simulink model "ProyectoGlobal_AyCD_Cantu_LagoTejo"  (R2021a)
settings: Solver=ode23  StartTime=0.0  StopTime=inf  MinStep=1e-4
values from neighbouring files (symbols this model uses):
  a_hMax = 0.75    [Datos_ProyectoGlobal_AyCD_Cantu_LagoTejo.m]    (also in Datos_v18.m; PID_calculado.mat)
  a_tMax = 0.8    [Datos_ProyectoGlobal_AyCD_Cantu_LagoTejo.m]    (also in Datos_v18.m; PID_calculado.mat)
  b_cx = 1e6    (= 1000000)    [Datos_ProyectoGlobal_AyCD_Cantu_LagoTejo.m]    (also in Datos_v18.m; PID_calculado.mat)
  b_cy = 1e7    (= 10000000)    [Datos_ProyectoGlobal_AyCD_Cantu_LagoTejo.m]    (also in Datos_v18.m; PID_calculado.mat)
  b_eq_h = ((b_hd + b_hm*(i_h^2))*2/(r_hd^2))    (= 31004.4444444)    [Datos_ProyectoGlobal_AyCD_Cantu_LagoTejo.m]    (also in Datos_v18.m; PID_calculado.mat)
  b_eq_t = ((b_td + b_tm*(i_t^2))/(r_td^2))    (= 21607.2)    [Datos_ProyectoGlobal_AyCD_Cantu_LagoTejo.m]    (also in Datos_v18.m; PID_calculado.mat)
  b_hb = 1e8    (= 100000000)    [Datos_ProyectoGlobal_AyCD_Cantu_LagoTejo.m]    (also in Datos_v18.m; PID_calculado.mat)
  b_hEb = 2.2e9    (= 2200000000)    [Datos_ProyectoGlobal_AyCD_Cantu_LagoTejo.m]    (also in Datos_v18.m; PID_calculado.mat)
  b_t = 90    [Datos_ProyectoGlobal_AyCD_Cantu_LagoTejo.m]    (also in Datos_v18.m; PID_calculado.mat)
  b_tb = 5e6    (= 5000000)    [Datos_ProyectoGlobal_AyCD_Cantu_LagoTejo.m]    (also in Datos_v18.m; PID_calculado.mat)
  b_tw = 3e3    (= 3000)    [Datos_ProyectoGlobal_AyCD_Cantu_LagoTejo.m]    (also in Datos_v18.m; PID_calculado.mat)
  b_wu = 150    [Datos_ProyectoGlobal_AyCD_Cantu_LagoTejo.m]    (also in Datos_v18.m; PID_calculado.mat)
  bah = M_eq_h*n_h*omega_h    [PID_Izaje_B.m]    (also in PID_calculado.mat = 387555.555556)
  bat = M_eq_t*n_t*omega_t    [PID_Carro_B.m]    (also in PID_calculado.mat = 270090)
  CI_h = 5    [Datos_ProyectoGlobal_AyCD_Cantu_LagoTejo.m]    (also in Datos_v18.m; PID_calculado.mat)
  CI_t = -16.25    [Datos_ProyectoGlobal_AyCD_Cantu_LagoTejo.m]    (also in Datos_v18.m; PID_calculado.mat)
  d_t = 1e-3    (= 0.001)    [Datos_ProyectoGlobal_AyCD_Cantu_LagoTejo.m]    (also in Datos_v18.m; PID_calculado.mat)
  g = 9.80665    [Datos_ProyectoGlobal_AyCD_Cantu_LagoTejo.m]    (also in Datos_v18.m; PID_calculado.mat)
  H_c = 2.5    [Datos_ProyectoGlobal_AyCD_Cantu_LagoTejo.m]    (also in Datos_v18.m; PID_calculado.mat)
  i_h = 22    [Datos_ProyectoGlobal_AyCD_Cantu_LagoTejo.m]    (also in Datos_v18.m; PID_calculado.mat)
  i_t = 30    [Datos_ProyectoGlobal_AyCD_Cantu_LagoTejo.m]    (also in Datos_v18.m; PID_calculado.mat)
  k_cy = 1.8e9    (= 1800000000)    [Datos_ProyectoGlobal_AyCD_Cantu_LagoTejo.m]    (also in Datos_v18.m; PID_calculado.mat)
  k_tw = 4.8e5    (= 480000)    [Datos_ProyectoGlobal_AyCD_Cantu_LagoTejo.m]    (also in Datos_v18.m; PID_calculado.mat)
  k_wu = 2.36e8    (= 236000000)    [Datos_ProyectoGlobal_AyCD_Cantu_LagoTejo.m]    (also in Datos_v18.m; PID_calculado.mat)
  Kd_bal = [-2.22044604925e-16 2.22044604925e-16 2.22044604925e-16 0 0 0 0 0 -2.22044604925e-16 0 2.22044604925e-16 -2.22044604925e-16 ... (296091 elements, 501x591)]    [Kp_Kd_balanceo.mat]    (also in PD_Balanceo.m = zeros(length(ML),length(L)))
  Kp_bal = [5.11381136401 5.1081388039 5.10248507909 5.09685008556 5.09123372013 5.08563588037 5.08005646467 5.07449537218 5.06895250283 5.06342775732 5.05792103709 5.05243224433 ... (296091 elements, 501x591)]    [Kp_Kd_balanceo.mat]    (also in PD_Balanceo.m = Kd_bal)
  ksah = M_eq_h*n_h*(omega_h^2)    [PID_Izaje_B.m]    (also in PID_calculado.mat = 922348.374575)
  ksat = M_eq_t*n_t*(omega_t^2)    [PID_Carro_B.m]    (also in PID_calculado.mat = 972648.108)
  ksiah = M_eq_h*n_h*(omega_h^3)    [PID_Izaje_B.m]    (also in PID_calculado.mat = 2195108.57705)
  ksiat = M_eq_t*n_t*(omega_t^3)    [PID_Carro_B.m]    (also in PID_calculado.mat = 3502700.36653)
  lim_xDer = 50    [Datos_ProyectoGlobal_AyCD_Cantu_LagoTejo.m]    (also in Datos_v18.m; PID_calculado.mat)
  lim_xDer_ult = 51    [Datos_ProyectoGlobal_AyCD_Cantu_LagoTejo.m]    (also in Datos_v18.m; PID_calculado.mat)
  lim_xIzq = -30    [Datos_ProyectoGlobal_AyCD_Cantu_LagoTejo.m]    (also in Datos_v18.m; PID_calculado.mat)
  lim_xIzq_ult = -31    [Datos_ProyectoGlobal_AyCD_Cantu_LagoTejo.m]    (also in Datos_v18.m; PID_calculado.mat)
  lim_yInf = -20    [Datos_ProyectoGlobal_AyCD_Cantu_LagoTejo.m]    (also in Datos_v18.m; PID_calculado.mat)
  lim_yInf_ult = -21    [Datos_ProyectoGlobal_AyCD_Cantu_LagoTejo.m]    (also in Datos_v18.m; PID_calculado.mat)
  lim_ySup = 40    [Datos_ProyectoGlobal_AyCD_Cantu_LagoTejo.m]    (also in Datos_v18.m; PID_calculado.mat)
  lim_ySup_ult = 41    [Datos_ProyectoGlobal_AyCD_Cantu_LagoTejo.m]    (also in Datos_v18.m; PID_calculado.mat)
  M_cMax = 50000    [Datos_ProyectoGlobal_AyCD_Cantu_LagoTejo.m]    (also in Datos_v18.m; PID_calculado.mat)
  M_cMin = 2000    [Datos_ProyectoGlobal_AyCD_Cantu_LagoTejo.m]    (also in Datos_v18.m; PID_calculado.mat)
  M_eq_h = (J_hd_hEb+J_hm_hb*i_h^2)*2/r_hd^2    (= 65137.7777778)    [Datos_ProyectoGlobal_AyCD_Cantu_LagoTejo.m]    (also in Datos_v18.m; PID_calculado.mat)
  M_l_max = 32500    [Datos_ProyectoGlobal_AyCD_Cantu_LagoTejo.m]    (also in Datos_v18.m; PID_calculado.mat)
  M_l_nom = 65000    [Datos_ProyectoGlobal_AyCD_Cantu_LagoTejo.m]    (also in Datos_v18.m; PID_calculado.mat)
  M_s = 15000    [Datos_ProyectoGlobal_AyCD_Cantu_LagoTejo.m]    (also in Datos_v18.m; PID_calculado.mat)
  M_t = 30000    [Datos_ProyectoGlobal_AyCD_Cantu_LagoTejo.m]    (also in Datos_v18.m; PID_calculado.mat)
  P_h_nom = 956.15e3    (= 956150)    [Datos_ProyectoGlobal_AyCD_Cantu_LagoTejo.m]    (also in Datos_v18.m; PID_calculado.mat)
  r_hd = 0.75    [Datos_ProyectoGlobal_AyCD_Cantu_LagoTejo.m]    (also in Datos_v18.m; PID_calculado.mat)
  r_td = 0.5    [Datos_ProyectoGlobal_AyCD_Cantu_LagoTejo.m]    (also in Datos_v18.m; PID_calculado.mat)
  T_hbMax = 5e4    (= 50000)    [Datos_ProyectoGlobal_AyCD_Cantu_LagoTejo.m]    (also in Datos_v18.m; PID_calculado.mat)
  T_hEbMax = 1.1e6    (= 1100000)    [Datos_ProyectoGlobal_AyCD_Cantu_LagoTejo.m]    (also in Datos_v18.m; PID_calculado.mat)
  T_hmMax = 2e4    (= 20000)    [Datos_ProyectoGlobal_AyCD_Cantu_LagoTejo.m]    (also in Datos_v18.m; PID_calculado.mat)
  T_tbMax = 5e3    (= 5000)    [Datos_ProyectoGlobal_AyCD_Cantu_LagoTejo.m]    (also in Datos_v18.m; PID_calculado.mat)
  T_tmMax = 3e3    (= 3000)    [Datos_ProyectoGlobal_AyCD_Cantu_LagoTejo.m]    (also in Datos_v18.m; PID_calculado.mat)
  tau_hm = 1e-3    (= 0.001)    [Datos_ProyectoGlobal_AyCD_Cantu_LagoTejo.m]    (also in Datos_v18.m; PID_calculado.mat)
  tau_tm = 1e-3    (= 0.001)    [Datos_ProyectoGlobal_AyCD_Cantu_LagoTejo.m]    (also in Datos_v18.m; PID_calculado.mat)
  v_hMax_0 = 3    [Datos_ProyectoGlobal_AyCD_Cantu_LagoTejo.m]    (also in Datos_v18.m; PID_calculado.mat)
  v_hMax_l = 1.5    [Datos_ProyectoGlobal_AyCD_Cantu_LagoTejo.m]    (also in Datos_v18.m; PID_calculado.mat)
  v_tMax = 4    [Datos_ProyectoGlobal_AyCD_Cantu_LagoTejo.m]    (also in Datos_v18.m; PID_calculado.mat)
  xc = [-28.75 -26.25 -23.75 -21.25 -18.75 -16.25 -13.75 -11.25 -8.75 -6.25 -3.75 -1.25 ... (32 elements, 1x32)]    [PID_calculado.mat]    (also in Perfil_Carga.m = -30+1.25:2.5:50-1.25)
  Y_sb = 15    [Datos_ProyectoGlobal_AyCD_Cantu_LagoTejo.m]    (also in Datos_v18.m; PID_calculado.mat)
  Y_t0 = 45    [Datos_ProyectoGlobal_AyCD_Cantu_LagoTejo.m]    (also in Datos_v18.m; PID_calculado.mat)
  yc = [0 0 0 2.5 0 2.5 0 2.5 0 0 0 0 ... (32 elements, 1x32)]    [PID_calculado.mat]    (also in Perfil_Carga.m = yc2)
undefined symbols (not defined in the file or in its folder): b_eq_td, M_eq_td
libraries: simulink x13
(part 2 of 2)

== system ProyectoGlobal_AyCD_Cantu_LagoTejo/Modelo Fisico Carro-Izaje-Carga/Carro/Carro y Cable de Carro ==
  theta : Inport
  F_hw : Inport  Port=2
  F_tw : Inport  Port=3
  1/M_t : Gain  Gain=1/M_t
  Gain : Gain  Gain=2
  Integrator : Integrator  InitialCondition=CI_t
  Integrator2 : Integrator
  Product : Product
  Sin : Trigonometry
  Sum1 : Sum  Inputs=++-
  b_t : Gain  Gain=b_t
  x_t : Outport
  d_x_t : Outport  Port=2
  wires:
  Sum1/1 -> 1/M_t/1
  Integrator2/1 -> d_x_t/1, b_t/1, Integrator/1
  theta/1 -> Sin/1
  Sin/1 -> Product/2
  F_hw/1 -> Gain/1
  Gain/1 -> Product/1
  Product/1 -> Sum1/2
  b_t/1 -> Sum1/3
  1/M_t/1 -> Integrator2/1
  Integrator/1 -> x_t/1
  F_tw/1 -> Sum1/1

== system ProyectoGlobal_AyCD_Cantu_LagoTejo/Modelo Fisico Carro-Izaje-Carga/Carro/Fuerza Cable Carro ==
  d_x_td : Inport
  d_x_t : Inport  Port=2
  x_td : Inport  Port=3
  x_t : Inport  Port=4
  Gain : Gain  Gain=k_tw
  Gain1 : Gain  Gain=b_tw
  Sum : Sum  Inputs=+|-
  Sum1 : Sum  Inputs=+|-
  Sum2 : Sum  Inputs=+|+
  F_tw : Outport
  wires:
  x_td/1 -> Sum/1
  Gain/1 -> Sum2/2
  Gain1/1 -> Sum2/1
  d_x_td/1 -> Sum1/1
  x_t/1 -> Sum/2
  Sum1/1 -> Gain1/1
  Sum2/1 -> F_tw/1
  Sum/1 -> Gain/1
  d_x_t/1 -> Sum1/2

== system ProyectoGlobal_AyCD_Cantu_LagoTejo/Modelo Fisico Carro-Izaje-Carga/Frenos/Freno Carro ==
  On_Off : Inport
  w_tm : Inport  Port=2
  Constant : Constant  Value=0
  Gain : Gain  Gain=-b_tb
  Saturation : Saturate  UpperLimit=T_tbMax  LowerLimit=-T_tbMax
  Switch : Switch  Criteria=u2 ~= 0
  T_tb : Outport
  wires:
  On_Off/1 -> Switch/2
  Constant/1 -> Switch/1
  w_tm/1 -> Gain/1
  Gain/1 -> Saturation/1
  Saturation/1 -> Switch/3
  Switch/1 -> T_tb/1

== system ProyectoGlobal_AyCD_Cantu_LagoTejo/Modelo Fisico Carro-Izaje-Carga/Frenos/Freno Emergencia Izaje ==
  On_Off : Inport
  w_hd : Inport  Port=2
  Constant : Constant  Value=0
  Gain : Gain  Gain=-b_hEb
  Saturation : Saturate  UpperLimit=T_hEbMax  LowerLimit=-T_hEbMax
  Switch : Switch  Criteria=u2 ~= 0
  T_hEb : Outport
  wires:
  On_Off/1 -> Switch/2
  Constant/1 -> Switch/1
  w_hd/1 -> Gain/1
  Gain/1 -> Saturation/1
  Saturation/1 -> Switch/3
  Switch/1 -> T_hEb/1

== system ProyectoGlobal_AyCD_Cantu_LagoTejo/Modelo Fisico Carro-Izaje-Carga/Frenos/Freno Izaje ==
  On_Off : Inport
  w_hm : Inport  Port=2
  Constant : Constant  Value=0
  Gain : Gain  Gain=-b_hb
  Saturation : Saturate  UpperLimit=T_hbMax  LowerLimit=-T_hbMax
  Switch : Switch  Criteria=u2 ~= 0
  T_hb : Outport
  wires:
  On_Off/1 -> Switch/2
  Constant/1 -> Switch/1
  w_hm/1 -> Gain/1
  Gain/1 -> Saturation/1
  Saturation/1 -> Switch/3
  Switch/1 -> T_hb/1

== system ProyectoGlobal_AyCD_Cantu_LagoTejo/Modelo Fisico Carro-Izaje-Carga/Izaje/Fuerza cable de Izaje ==
  l : Inport
  l_h : Inport  Port=2
  d_l : Inport  Port=3
  d_l_h : Inport  Port=4
  Gain6 : Gain  Gain=2
  Gain7 : Gain  Gain=2
  Product2 : Product
  Product3 : Product
  Saturation : Saturate  UpperLimit=inf  LowerLimit=0
  Sum2 : Sum  Inputs=+|-
  Sum6 : Sum  Inputs=+|+
  Sum7 : Sum  Inputs=+|-
  b_w y k_w : Subsystem
  F_hw : Outport
  wires:
  Sum2/1 -> Gain6/1
  l_h/1 -> Sum2/2, b_w y k_w/1(l_h)
  Gain6/1 -> Product2/1
  b_w y k_w/2(K_w) -> Product2/2
  Sum7/1 -> Gain7/1
  Gain7/1 -> Product3/1
  b_w y k_w/1(b_w) -> Product3/2
  Product2/1 -> Sum6/2
  Product3/1 -> Sum6/1
  Sum6/1 -> Saturation/1
  l/1 -> Sum2/1
  d_l_h/1 -> Sum7/2
  d_l/1 -> Sum7/1
  Saturation/1 -> F_hw/1

== system ProyectoGlobal_AyCD_Cantu_LagoTejo/Modelo Fisico Carro-Izaje-Carga/Izaje/Izaje Eje Rapido-Lento ==
  F_hw : Inport
  T_hm : Inport  Port=2
  T_hEb : Inport  Port=3
  T_hb : Inport  Port=4
  1/M_eq_h : Gain  Gain=1/M_eq_h
  Constant : Constant  Value=Y_t0
  Gain : Gain  Gain=-1
  Gain1 : Gain  Gain=1/r_hd
  Gain2 : Gain  Gain=i_h/r_hd
  Integrator2 : Integrator
  Integrator3 : Integrator  InitialCondition=CI_h
  Sum : Sum  Inputs=|++
  Sum1 : Sum  Inputs=-+-
  Sum2 : Sum  Inputs=|++
  Sum3 : Sum  Inputs=+|-
  b_eq_h : Gain  Gain=b_eq_h
  l_h : Outport
  d_l_h : Outport  Port=2
  x_hd : Outport  Port=3
  d_x_hd : Outport  Port=4
  wires:
  Integrator2/1 -> d_x_hd/1, Gain/1, b_eq_h/1, Integrator3/1
  1/M_eq_h/1 -> Integrator2/1
  b_eq_h/1 -> Sum1/3
  F_hw/1 -> Sum1/1
  T_hm/1 -> Sum/1
  T_hEb/1 -> Gain1/1
  T_hb/1 -> Sum/2
  Constant/1 -> Sum3/1
  Sum3/1 -> l_h/1
  Integrator3/1 -> x_hd/1, Sum3/2
  Sum1/1 -> 1/M_eq_h/1
  Sum/1 -> Gain2/1
  Gain/1 -> d_l_h/1
  Sum2/1 -> Sum1/2
  Gain1/1 -> Sum2/2
  Gain2/1 -> Sum2/1

== system ProyectoGlobal_AyCD_Cantu_LagoTejo/Modelo Fisico Carro-Izaje-Carga/Limites de operacion/Límites de Carro ==
  x_t : Inport
  Constant : Constant  Value=lim_xIzq_ult
  Constant1 : Constant  Value=lim_xIzq
  Constant2 : Constant  Value=lim_xDer_ult
  Constant3 : Constant  Value=lim_xDer
  Equal : RelationalOperator  Operator=<=  OutDataTypeStr=boolean  RndMeth=Simplest
  Equal1 : RelationalOperator  Operator=<=  OutDataTypeStr=boolean  RndMeth=Simplest
  Equal2 : RelationalOperator  OutDataTypeStr=boolean  RndMeth=Simplest
  Equal3 : RelationalOperator  OutDataTypeStr=boolean  RndMeth=Simplest
  fc_izq_norm : Outport
  fc_izq_ult : Outport  Port=2
  fc_der_norm : Outport  Port=3
  fc_der_ult : Outport  Port=4
  wires:
  Constant/1 -> Equal1/2
  Constant1/1 -> Equal/2
  Constant3/1 -> Equal2/2
  Constant2/1 -> Equal3/2
  Equal1/1 -> fc_izq_ult/1
  Equal3/1 -> fc_der_ult/1
  Equal2/1 -> fc_der_norm/1
  x_t/1 -> Equal2/1, Equal3/1, Equal1/1, Equal/1
  Equal/1 -> fc_izq_norm/1

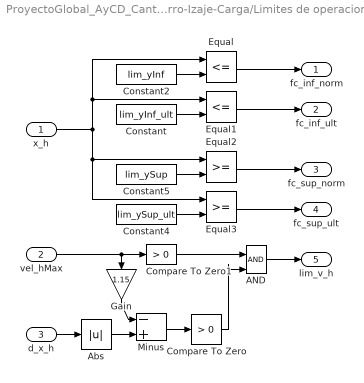
== system ProyectoGlobal_AyCD_Cantu_LagoTejo/Modelo Fisico Carro-Izaje-Carga/Limites de operacion/Subsystem1 ==
  x_h : Inport
  vel_hMax : Inport  Port=2
  d_x_h : Inport  Port=3
  AND : Logic  IconShape=distinctive  AllPortsSameDT=off  OutDataTypeStr=boolean
  Abs : Abs
  Compare To Zero : simulink/Logic and Bit Operations/Compare To Zero  relop=>  OutDataTypeStr=boolean
  Compare To Zero1 : simulink/Logic and Bit Operations/Compare To Zero  relop=>  OutDataTypeStr=boolean
  Constant : Constant  Value=lim_yInf_ult
  Constant2 : Constant  Value=lim_yInf
  Constant4 : Constant  Value=lim_ySup_ult
  Constant5 : Constant  Value=lim_ySup
  Equal : RelationalOperator  Operator=<=  OutDataTypeStr=boolean  RndMeth=Simplest
  Equal1 : RelationalOperator  Operator=<=  OutDataTypeStr=boolean  RndMeth=Simplest
  Equal2 : RelationalOperator  OutDataTypeStr=boolean  RndMeth=Simplest
  Equal3 : RelationalOperator  OutDataTypeStr=boolean  RndMeth=Simplest
  Gain : Gain  Gain=1.15
  Minus : Sum  Inputs=-+
  fc_inf_norm : Outport
  fc_inf_ult : Outport  Port=2
  fc_sup_norm : Outport  Port=3
  fc_sup_ult : Outport  Port=4
  lim_v_h : Outport  Port=5
  wires:
  Abs/1 -> Minus/2
  vel_hMax/1 -> Gain/1, Compare To Zero1/1
  d_x_h/1 -> Abs/1
  Minus/1 -> Compare To Zero/1
  Constant4/1 -> Equal3/2
  Equal1/1 -> fc_inf_ult/1
  Equal/1 -> fc_inf_norm/1
  Constant/1 -> Equal1/2
  Equal3/1 -> fc_sup_ult/1
  Constant5/1 -> Equal2/2
  Equal2/1 -> fc_sup_norm/1
  x_h/1 -> Equal2/1, Equal3/1, Equal1/1, Equal/1
  Constant2/1 -> Equal/2
  AND/1 -> lim_v_h/1
  Compare To Zero1/1 -> AND/1
  Compare To Zero/1 -> AND/2
  Gain/1 -> Minus/1

== system ProyectoGlobal_AyCD_Cantu_LagoTejo/Modelo Fisico Carro-Izaje-Carga/theta y l/Subsystem ==
  x_l : Inport
  d_x_l : Inport  Port=2
  x_t : Inport  Port=3
  d_x_t : Inport  Port=4
  y_l : Inport  Port=5
  d_y_l : Inport  Port=6
  l : Inport  Port=7
  Constant : Constant  Value=Y_t0
  Divide : Product  Inputs=*/
  Product : Product
  Product1 : Product
  Sum{,1..3} (4 alike) : Sum  Inputs=+|-
  d_l : Outport
  wires:
  l/1 -> Divide/2
  Product/1 -> Sum/1
  Product1/1 -> Sum/2
  x_l/1 -> Sum1/1
  x_t/1 -> Sum1/2
  Sum1/1 -> Product/1
  d_x_l/1 -> Sum2/1
  d_x_t/1 -> Sum2/2
  Sum2/1 -> Product/2
  d_y_l/1 -> Product1/1
  Constant/1 -> Sum3/1
  y_l/1 -> Sum3/2
  Sum3/1 -> Product1/2
  Sum/1 -> Divide/1
  Divide/1 -> d_l/1

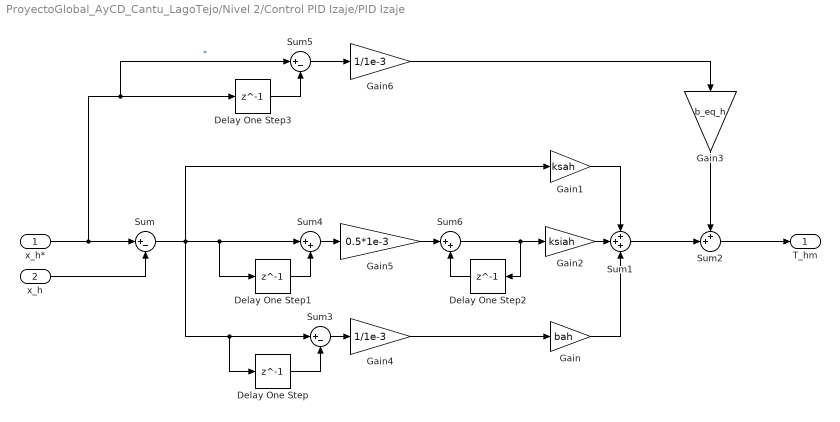
== system ProyectoGlobal_AyCD_Cantu_LagoTejo/Nivel 2/Control PID Izaje/PID Izaje ==
  x_h* : Inport
  x_h : Inport  Port=2
  Delay One Step{,1..3} (4 alike) : Delay  DelayLength=1  SampleTime=1e-3
  Gain : Gain  Gain=bah
  Gain1 : Gain  Gain=ksah
  Gain2 : Gain  Gain=ksiah
  Gain3 : Gain  Gain=b_eq_h
  Gain4 : Gain  Gain=1/1e-3
  Gain5 : Gain  Gain=0.5*1e-3
  Gain6 : Gain  Gain=1/1e-3
  Sum : Sum  Inputs=|+-
  Sum1 : Sum  Inputs=+++
  Sum2 : Sum  Inputs=++|
  Sum3 : Sum  Inputs=|+-
  Sum4 : Sum  Inputs=|++
  Sum5 : Sum  Inputs=|+-
  Sum6 : Sum  Inputs=|++
  T_hm : Outport
  wires:
  Gain2/1 -> Sum1/2
  Gain1/1 -> Sum1/1
  Gain/1 -> Sum1/3
  x_h/1 -> Sum/2
  Gain3/1 -> Sum2/1
  Sum1/1 -> Sum2/2
  Sum2/1 -> T_hm/1
  Sum3/1 -> Gain4/1
  Gain4/1 -> Gain/1
  Delay One Step/1 -> Sum3/2
  Sum4/1 -> Gain5/1
  Delay One Step1/1 -> Sum4/2
  Sum/1 -> Delay One Step1/1, Sum4/1, Delay One Step/1, Sum3/1, Gain1/1
  Sum6/1 -> Gain2/1, Delay One Step2/1
  Gain6/1 -> Gain3/1
  Delay One Step3/1 -> Sum5/2
  Sum5/1 -> Gain6/1
  Delay One Step2/1 -> Sum6/2
  Gain5/1 -> Sum6/1
  x_h*/1 -> Sum/1, Sum5/1, Delay One Step3/1  "*"

== system ProyectoGlobal_AyCD_Cantu_LagoTejo/Modelo Fisico Carro-Izaje-Carga/Izaje/Fuerza cable de Izaje/b_w y k_w ==
  l_h : Inport
  Constant1 : Constant  Value=k_wu
  Constant2 : Constant  Value=110
  Constant3 : Constant  Value=b_wu
  Constant4 : Constant  Value=110
  Divide2 : Product  Inputs=*/
  Gain1 : Gain  Gain=2
  Gain6 : Gain  Gain=2
  Product : Product
  Sum1 : Sum  Inputs=|++
  Sum2 : Sum  Inputs=|++
  b_w : Outport
  K_w : Outport  Port=2
  wires:
  Sum2/1 -> Product/2
  Gain6/1 -> Sum2/1
  Constant3/1 -> Product/1
  Constant4/1 -> Sum2/2
  Product/1 -> b_w/1
  l_h/1 -> Gain6/1, Gain1/1
  Constant1/1 -> Divide2/1
  Constant2/1 -> Sum1/2
  Sum1/1 -> Divide2/2
  Gain1/1 -> Sum1/1
  Divide2/1 -> K_w/1

== matlab function ProyectoGlobal_AyCD_Cantu_LagoTejo/MATLAB Function1 ==
  data: clock input; BRK_t input; BRK_h input; ON_OFF input; sist_OK input; Manual input; Ciclo input; max_masa input; Tension_hw input; TLK input; Balanceo input; manual_auto input; ml_medida input; xc input; yc input; graficar input; x_l input; y_l input; x_td input
function grafico_puerto(clock, BRK_t, BRK_h, ON_OFF, sist_OK, Manual, Ciclo, max_masa, Tension_hw, TLK, Balanceo, manual_auto, ml_medida, xc, yc, graficar, x_l, y_l, x_td)
if(graficar==1)
    alt_txt = 14;   color_cont = "#90AC50";
    fh = figure(100);
    % fh.WindowState = 'maximized';
    clf(fh);
    title('Simulación Visual en Tiempo "Real"'),    grid on
    rectangle('Position',[-30, 46, 80, 4],'FaceColor', '#EEEEEE','EdgeColor','k')
    rectangle('Position',[-30, -20, 30, 20],'FaceColor', 'w')
    line([-30 0],[-0.5 -0.5],'Color','black','LineWidth', 5)                    %%% Muelle
    rectangle('Position',[-0.5, 0, 0.5, 15],'FaceColor','black');               %%% Sill Beam
    rectangle('Position',[0.5, -20, 49.5, 25],'EdgeColor','b','LineWidth', 1.5);%%% Barco
    rectangle('Position',[-30, 45, 80, 2],'FaceColor',[0.8 0.8 1]);             %%% Grúa
    rectangle('Position',[x_l-1.25,y_l,2.5,0.5],'FaceColor','k');               %%% Spreader
    rectangle('Position',[x_td-2.5, 45, 5, 2],'FaceColor','k');              %%% Carro
    line([x_l x_td], [y_l 45],'Color','black','LineWidth',2)                 %%% Cable

    for i=1:length(yc)                  %%% Perfil de Carga
        if (xc(i)<2.5)                  %%% Lado de Muelle
            % rectangle('Position',[xc(i)-1.25,0,2.5,yc(i)],'FaceColor', color_cont,'LineWidth', 0.3);
            cant = abs(yc(i)/2.5);
            if cant>0
                for j=1:cant
                    yc_cant_bottom = 2.5*(j-1);
                    rectangle('Position',[xc(i)-1.25,yc_cant_bottom,2.5,2.5],'FaceColor', color_cont,'LineWidth', 0.3);
                end
            end
        elseif(xc(i)>2.5 && xc(i)<47.5) %%% Lado de Barco
            % rectangle('Position',[xc(i)-1.25,-20,2.5,yc(i)+20],'FaceColor', color_cont,'LineWidth', 0.3);
            cant = abs(yc(i)+20)/2.5;
            if cant>0
                for j=1:cant
                    yc_cant_bottom = 2.5*(j-1) - 20;
                    rectangle('Position',[xc(i)-1.25,yc_cant_bottom,2.5,2.5],'FaceColor', color_cont,'LineWidth', 0.3);
                end
            end
        end
    end

    txt000 = {'Tiempo: ', clock};       %%% Tiempo de Ejecución "Real"
    text(-10, -3.5, txt000,'FontSize', alt_txt)
    
%     if (BRK_t==0)                       %%% Cartel Freno Carro
%         txt = {'Freno Carro'};
%         text(-10, -10, txt,'FontSize', alt_txt,'Color','#FF0000')
%     end
%     if (BRK_h==0)                       %%% Cartel Freno Izaje
%         txt = {'Freno Izaje'};
%         text(-10, -17, txt,'FontSize', alt_txt,'Color','#FF0000')
%     end

    if(ON_OFF)                          %%% Cartel de ON - OFF
        txt00 = {'ON: Encendido'};
        text(-30,48.5,txt00,'FontSize',alt_txt,'Color',"#00AA00")
    else
        txt00 = {'OFF: APAGADO'};
        text(-30,48.5,txt00,'FontSize',alt_txt,'Color',"#FF0000")
    end
    
    txt = {'Masa: ', ml_medida};               %%% Cartel de Masa Total en Spreader
    text(-29.75,-17,txt,'FontSize',alt_txt)

    if (TLK)                                   %%% Cartel de Cargado/Sin Carga/SOBRECARGA
        rectangle('Position',[x_l-1.25,y_l-2.5,2.5,2.5],'FaceColor', color_cont,'LineWidth', 0.3); %carga
        if(ml_medida > 15000)
            if (max_masa)
                txt01 = {'SOBRECARGA'};
                text(-20,-17,txt01,'Color','red','FontSize',alt_txt+4)
            else
                txt01 = {'Cargado'};
                text(-20,-17,txt01,'Color',"#00AA00",'FontSize',alt_txt+2)
            end
        else
            txt01 = {'Sin Carga'};
            text(-20,-17,txt01,'Color',"#CB7A00",'FontSize',alt_txt+2)
        end
    end

    if (Manual)                       %%% Cartel de Modo de Control
        txt02 = {'Manual'};
        text(-15, 48.5,txt02,'FontSize', alt_txt)
    else
        if (manual_auto)
            txt02 = {'Automático'};
            text(-15, 48.5,txt02,'FontSize',alt_txt)
        else
            txt02 = {'Manual'};
            text(-15, 48.5,txt02,'FontSize',alt_txt)
        end
    end

    if (Balanceo)                       %%% Cartel de Control de Balanceo
        txt03 = {'Balanceo: ON'};
        text(-4, 48.5, txt03,'FontSize',alt_txt,'Color',"#00AA00")
    else
        txt03 = {'Balanceo: OFF'};
        text(-4, 48.5,txt03,'FontSize', alt_txt,'Color','#FF0000')
    end

    if (Tension_hw)                     %%% Cartel de Spreader Apoyado o Suspendido
        txt04 = {'Suspendido'};
        text(10,48.5,txt04,'FontSize', alt_txt)
    else
        txt04 = {'Apoyado'};
        text(10,48.5,txt04,'FontSize', alt_txt)
    end

    if (Ciclo)                          %%% Cartel de Tipo de Ciclo
        txt05 = {'Ciclo Doble'};
        text(22,48.5,txt05,'FontSize', alt_txt)
    else
        txt05 = {'Ciclo Simple'};
        text(22,48.5,txt05,'FontSize', alt_txt)
    end
    
    if (sist_OK==0)                 %%% Cartel de EMERGENCIA (botón)
        txt7 = {'EMERGENCIA'};
        rectangle('Position',[34.5, 47, 15.5, 3],'FaceColor', 'red')
        text(35.5,48.5,txt7,'FontSize', alt_txt+6,'Color',"w")
    else
        txt7 = {'OK'};
        rectangle('Position',[34.5, 47, 15.5, 3],'FaceColor', "#00FF00")
        text(41,48.5,txt7,'FontSize', alt_txt+6,'Color',"k")
    end
  
    txt1 = {'Carro (X): ',x_td};                %%% Posiciones del Carro
    text(-29.75,-3.5,txt1,'FontSize',alt_txt)
    txt1 = {'Carro (Y): ',45};
    text(-20,-3.5,txt1,'FontSize',alt_txt)
    txt1 = {'Spreader (X): ',x_l};              %%% Posiciones del Spreader
    text(-29.75,-10,txt1,'FontSize',alt_txt)
    txt1 = {'Spreader (Y): ',y_l};
    text(-20,-10,txt1,'FontSize',alt_txt)
end
end

== matlab function ProyectoGlobal_AyCD_Cantu_LagoTejo/Modelo Fisico Carro-Izaje-Carga/Modos de Contacto/MATLAB Function1 ==
  data: Susp input; Y_c0 output size=1; x_l input; Yc input; Xc input; TLK input; TLKold input; yc_act_old input size=[1 32]; yc_act output size=[1 32]; change output size=1
function [Y_c0,yc_act,  change] = yc_actual(Susp,x_l,Yc,Xc,TLK,TLKold,yc_act_old)
%Susp: modo de contacto (1 suspendido , 0 apoyado)
change=0;

%yc_act = zeros(1,length(yc));
%Posicionamiento de container en el plano
idx=1;

for i=1:length(Xc)
    if ((x_l>=(Xc(i)-1.25))&&(x_l<(Xc(i)+1.25)))
        idx = i;
    end
end

if(yc_act_old == Yc)
    %Cierra el Twistlock -> Container tomado(Se quita del suelo)
    if((TLK==1) && (TLKold==0) && (Susp==0))
        
        if(x_l>2.5 && x_l<47.5)
            
            if(Yc(idx)>-20 )
                Yc(idx) = Yc(idx) - 2.5;
            end
            yc_act = Yc;
            Y_c0 = yc_act(idx);
            change=1;
            
        elseif(x_l>-37.5 && x_l <-2.5)
            
            if(Yc(idx)>0)
                Yc(idx) = Yc(idx) - 2.5;
            end
            yc_act = Yc;
            Y_c0 = yc_act(idx);
            change=1;
            
        end
        
        %Abre el Twistlock -> Container posicionado y soltado(Se agrega al suelo)
    elseif((TLK==0) && (TLKold==1) && (Susp==0))
        if(Yc(idx)<32.5 )
            Yc(idx) = Yc(idx) + 2.5;
        end
        yc_act = Yc;
        Y_c0 = yc_act(idx);
        change=1;
    else
        change=0;
    end
    
end




yc_act = Yc;
Y_c0 = yc_act(idx);
end

== stateflow chart ProyectoGlobal_AyCD_Cantu_LagoTejo/Nivel 1 ==
  settings: updateMethod=DISCRETE  sampleTime=1e-3
  state HEARTBEAT [parallel]
    entry:
    WD=1;
    settings: executionOrder=2
    state ALTO
      WD=1;
    state BAJO
      WD=0;
    ALTO -> BAJO : after(50,msec)
    (default) -> ALTO
    BAJO -> ALTO : after(50,msec)
  state NIVEL_1 [parallel]
    settings: executionOrder=1
    state ENCENDIDO
      state TWISTLOCKS [parallel]
        settings: executionOrder=6
        state ASCENSO_LENTO
          entry:
          pesaje_cont = 1;
          manual_auto=1;
          cargado=1;
          vel_h=0.5;
        state ESTABILIZACION
          entry:
          vel_h = 0
        state VACIO %TLK_Off
          entry:
          vel_hMax=v_hMax_0;
          m_l=M_s;
          cargado=0;
          max_masa = 0;
          m_l_calc =0;
          pesaje_cont = 0;
        state CALC_MASA
          entry:
          m_l_calc = abs(F_hw*2/g)
          manual_auto = 0;
        state CARGADO %TLK_On
          entry:
          if (m_l_calc <= M_l_max)
          vel_hMax = v_hMax_0;
          elseif (m_l_calc > M_l_max && m_l < M_l_nom)
          vel_hMax = P_h_nom / (m_l_calc*g);
          elseif (m_l_calc >= M_l_nom)
          vel_hMax = v_hMax_l;
          end
          if((m_l_calc-M_s)>M_cMax)
          max_masa=1;
          end
          m_l=m_l_calc;
          pesaje_cont = 0;
        VACIO %TLK_Off -> ASCENSO_LENTO : [(sistOK==1)&&(TLK==1)&&(F_hw<=0)]
        ASCENSO_LENTO -> ESTABILIZACION : [(F_hw>0)]
        ESTABILIZACION -> CALC_MASA : after(5,sec)
        (default) -> VACIO %TLK_Off
        CALC_MASA -> CARGADO %TLK_On
        CARGADO %TLK_On -> VACIO %TLK_Off : [(TLK==0)&&(F_hw<=0)]
      state MANUAL_AUTO [parallel]
        entry:
        etapaDoble=0;
        ida=1;
        vuelta=0;
        settings: executionOrder=2
        state MODO_AUTOMATICO
          entry:
          manual_auto=1;
          Xsafe=CI_t; inicio_t=x_td;
          if ((Ciclo_Doble==1)&&(etapaDoble==1))
          Y_max_barco=Ymax_b(Yc,carril_finDoble)+2;
          Ysafe=Y_max_barco+5;
          elseif (etapaDoble==0)
          Y_max_barco = Ymax_b(Yc,carril_fin)+2;
          Ysafe=Y_max_barco+5;
          end
          lim_m2b=X_LIM(x_td,Xfin,Y_max_barco,Ysafe);
          state TRASLACION_AUTOMATICA [parallel]
            entry:
            settings: executionOrder=1
            state Mov_Traslacion
              entry:
              traslacion_calc(inicio_t,fin_t);
              vel_t = d_x_t;
              tx = 0;
              if ((Ciclo_Doble==1)&&(etapaDoble==0))
              etapaDoble=1;
              elseif ((Ciclo_Doble==1)&&(etapaDoble==1))
              etapaDoble=2;
              elseif ((Ciclo_Doble==1)&&(etapaDoble==2))
              etapaDoble=0;
              end
              during:
              if(after(d_t,sec))
              trasladar(inicio_t,fin_t,d_t);
              end
            state Inicio_Traslacion
            Inicio_Traslacion -> Mov_Traslacion [order 1] : [(lado == 0)&&(x_hd >=Y_sb-5)]
                | {fin_t=Xfin}
            (default) -> Inicio_Traslacion
            Inicio_Traslacion -> Mov_Traslacion [order 2] : [(lado == 1)&&(Ciclo_Doble==1)&&(etapaDoble==1)&&(x_hd >=Y_max_barco-2.5)]
                | {fin_t=XfinDoble;}
            Inicio_Traslacion -> Mov_Traslacion [order 3] : [(lado == 1)&&(x_hd >=Y_max_barco-2.5)]
                | {fin_t=Xsafe}
          state IZAJE_AUTOMATICO [parallel]
            entry:
            settings: executionOrder=2
            state Inicio_Izaje
              entry:
              vel_h = 0;
            state Mov_Izaje
              entry:
              izaje_calc(inicio_h,fin_h);
              vel_h = d_x_h;
              ty = 0;
              end
              during:
              if(after(d_t,sec))
              izar(inicio_h,fin_h,d_t)
              end
            Inicio_Izaje -> Mov_Izaje [order 4] : [(ida==1)&&(ascenso==1)&&(x_td >=lim_m2b-3)]
                | { inicio_h=x_hd; fin_h=Y_max_barco-4;ascenso=0;vuelta=1;ida=0}
            Inicio_Izaje -> Mov_Izaje [order 5] : [(vuelta==1)&&(ascenso==1)&&(x_td <=3)]
                | { inicio_h=x_hd; fin_h=Y_max_muelle-1;ascenso=0;vuelta=0;ida=1}
            (default) -> Inicio_Izaje
            Inicio_Izaje -> Mov_Izaje [order 3] : [(lado==1)&&(ascenso==1)&&(etapaDoble==2)&&(x_td >=XfinDoble-4)&&(x_td <=XfinDoble+0.5)]
                | { inicio_h=x_hd; fin_h=Y_max_barco-4;ascenso=0}
            Inicio_Izaje -> Mov_Izaje [order 2] : [(ascenso==0)&&(cargado==1)]{ inicio_h=x_hd; fin_h=Ysafe;ascenso=1}
            Inicio_Izaje -> Mov_Izaje [order 1] : [(ascenso==0)&&(cargado==0)]{ inicio_h=x_hd; fin_h=Ysafe-H_c;ascenso=1}
            Mov_Izaje -> Inicio_Izaje [order 2] : [(ascenso==0)&&(x_hd<=fin_h)]
            Mov_Izaje -> Inicio_Izaje [order 1] : [(ascenso==1)&&(x_hd>=fin_h-1)]
        state MODO_MANUAL
          entry:
          if(pesaje_cont == 0)
          manual_auto = 0;
          end
          during:
          [Xfin, XfinDoble] = carril2x(carril_fin, carril_finDoble, Xc);
        MODO_AUTOMATICO -> MODO_MANUAL : [(Manual==1) || ((lado==0)&&(x_hd<=Y_max_muelle)) || ((lado==1)&&(x_hd<=Y_lim_barco)) || (sistOK==0)||(in_izaje_on==1)||(in_carro_on==1)]
            | {vel_h = 0;vel_t = 0;}
        (default) -> MODO_MANUAL
        MODO_MANUAL -> MODO_AUTOMATICO : [(Manual==0)&&(((lado==0)&&(x_hd>Y_max_muelle))||((lado==1)&&(x_hd>Y_lim_barco)))&&(sistOK==1)]
      state POSICION_ACTUAL [parallel]
        settings: executionOrder=1
        state MUELLE
          entry:
          Y_max_muelle=8;
          Y_lim_barco = 15;
          lado=0;
        state BARCO
          entry:
          lado=1;
          Y_lim_barco = 15;
        MUELLE -> BARCO : [x_td>0]
        (default) -> MUELLE
        BARCO -> MUELLE : [x_td<=0]
      state CONTROL_DE_BALANCEO [parallel]
        settings: executionOrder=4
        state DESACTIVADO
          entry:
          Balanceo = 0;
        state ACTIVADO
          entry:
          Balanceo = 1;
        DESACTIVADO -> ACTIVADO : [(Manual==0)||(Balanceo_ctrl==1)]
        (default) -> ACTIVADO
        ACTIVADO -> DESACTIVADO : [(Manual==1)&&(Balanceo_ctrl==0)]
      state FRENO_DE_CARRO [parallel]
        settings: executionOrder=5
        state BRKt_DESACTIVADO
          entry:
          BRK_t=1;
        state BRKt_ACTIVADO
          entry:
          BRK_t=0;
        BRKt_DESACTIVADO -> BRKt_ACTIVADO : [(ON_OFF==0||(vel_t_on==0))]
        (default) -> BRKt_ACTIVADO
        BRKt_ACTIVADO -> BRKt_DESACTIVADO : [(ON_OFF==1)&&(vel_t_on==1)]
      state FRENO_DE_IZAJE [parallel]
        settings: executionOrder=3
        state BRKh_DESACTIVADO
          entry:
          BRK_h=1;
        state BRKh_ACTIVADO
          entry:
          BRK_h=0;
        BRKh_ACTIVADO -> BRKh_DESACTIVADO : [(ON_OFF==1)&&(vel_h_on==1)]
        (default) -> BRKh_ACTIVADO
        BRKh_DESACTIVADO -> BRKh_ACTIVADO : [(ON_OFF==0)||(vel_h_on==0)]
    state APAGADO
      during:
      BRK_t=0;
      BRK_h=0;
      m_l=M_s;
      manual_auto=0;
      max_masa=0;
      vel_h=0;
      vel_t=0;
      cargado=0;
    state FIN_DE_CARRERA
      entry:
      manual_auto=0;
      Balanceo = 0;
    state EMERGENCIA_N0
      during:
      Balanceo = 0;
      manual_auto=0;
      BRK_t=0;
      BRK_h=0;
      vel_h=0;
      vel_t=0;
    (default) -> APAGADO
    ENCENDIDO -> FIN_DE_CARRERA [order 2] : [(fc_izq_norm == 1) || (fc_der_norm ==1)]
        | {vel_t = 0}
    ENCENDIDO -> FIN_DE_CARRERA [order 3] : [(fc_inf_norm == 1) || (fc_sup_norm == 1)]
        | {vel_h = 0}
    FIN_DE_CARRERA -> ENCENDIDO [order 1] : [(ON_OFF==0)]
    APAGADO -> ENCENDIDO : [(ON_OFF==1)]
    FIN_DE_CARRERA -> ENCENDIDO [order 2] : [(fc_izq_norm==0)&&(fc_der_norm==0)&&(fc_inf_norm==0)&&(fc_sup_norm==0)&&(Manual==1)&&sistOK==1]
    ENCENDIDO -> APAGADO [order 1] : [(ON_OFF==0)]
    ENCENDIDO -> EMERGENCIA_N0 [order 4] : [BTN_EMERGENCIA==1]
  data: carrilFin function_input; carrilFinDoble function_input; Xcarga function_input; X_fin function_output; X_finDoble function_output; x_ini function_input; x_fin function_input; y_ini function_input; y_fin function_input; X function_output; x_ini function_input; x_fin function_input; x_ini function_input; x_fin function_input; delta_t function_input; y_ini function_input; y_fin function_input; y_ini function_input; y_fin function_input; delta_t function_input; Ycarga function_input size=[1 32]; carrilFin function_input size=1; YmaxBarco function_output size=1; in_izaje_on input; in_carro_on input; TLK input; H_c parameter double; M_s parameter double; BRK_h output size=1; Balanceo output size=1; vel_h_on input; Balanceo_ctrl input; ON_OFF input; sistOK input; vel_t_on input; x_td input; x_hd input; v_hMax_0 parameter; v_tMax parameter; F_hw input; Manual input; BTN_EMERGENCIA input; Ciclo_Doble input; fc_izq_norm input; fc_der_norm input; fc_inf_norm input; fc_sup_norm input; manual_auto output size=1; BRK_t output size=1; d_x_h input; d_x_t input; Yc input; M_cMax parameter; m_l output size=1; g parameter double; a_hMax parameter; a_tMax parameter; traj_h local; traj_t local; Yfin local double; Xini local double; Yini local double; vel_h output size=1; xrest local; d_t parameter; dx local; dy local; yrest local; ty local; M_l_nom parameter; P_h_nom parameter; v_hMax_l parameter; M_l_max parameter; vel_hMax output size=1; t1x local; t2x local; Dx local; tx local; vel_t output size=1; vx local; t1y local; Dy local; m_l_calc local; ty_tot local; t2y local; tstable1 local; tstable2 local; pesaje_cont local =0; x0 local; x2 local; y3 local; x4 local; y4 local; x1 local; y0 local; x3 local; y2 local; y1 local; desp_y local; desp_x local; vy local; x6 local; y6 local; x5 local; y5 local; lado local; x3_cd local; lim_b2m local; etapaDoble local; lim_m2b local; Ysafe local =0; Y_max_barco local size=1 =0; cargado output size=1; cont_bit local; WD output size=1; fin_h local; fin_t local; inicio_h local; inicio_t local; Xsafe local; Y_max local; Xc input; Y_max_muelle local; max_masa output size=1; carril_fin input; carril_finDoble input; XfinDoble local; Xfin local; etapaDoble_h local; ascenso local =0; CI_t parameter; Y_sb parameter; ida local; vuelta local; YsafeDoble local; Y_maxDoble local; Y_lim_barco local
  function [X_fin, X_finDoble] = carril2x(carrilFin, carrilFinDoble, Xcarga):
    | function [X_fin, X_finDoble] = carril2x(carrilFin, carrilFinDoble, Xcarga)
    | offsetCarrilesBarco = 13; % Total carriles:32 - carriles en barco:18 - carril final:1 =13
    | 
    | X_fin = Xcarga(carrilFin + offsetCarrilesBarco);
    | X_finDoble = Xcarga(carrilFinDoble + offsetCarrilesBarco);
    | end
  function X = X_LIM(x_ini,x_fin,y_ini,y_fin):
    | function X = X_LIM(x_ini,x_fin,y_ini,y_fin)
    | 
    | D_h = abs(y_fin - y_ini);     
    | 
    | T1_h = (vel_hMax - d_x_h)/a_hMax;    
    | T3_h = abs(vel_hMax/a_hMax);      
    | 
    | D1_h = d_x_h * T1_h + 0.5 * a_hMax * T1_h*T1_h;   
    | D3_h =   vel_hMax * T3_h - 0.5 * a_hMax * T3_h*T3_h;   
    | 
    | if ((D1_h + D3_h) <= D_h)
    |     y_rest = D_h - (D1_h + D3_h); 
    |     T2_h = T1_h + y_rest / vel_hMax;   
    |     Vy = vel_hMax;                  
    |     Ttot = T2_h + T3_h;       
    | else
    |     Vy = sqrt(a_hMax * D_h);   
    |     T3_h = Vy / a_hMax;       
    |     T2_h = T3_h - abs(d_x_h/a_hMax);
    |     Ttot = T2_h + T3_h;       
    | end
    | 
    | 
    | T3_t = abs(v_tMax/a_tMax);
    | 
    | if(Ttot>T3_t)
    |     A_rect = (Ttot - T3_t)*v_tMax;
    |     A_triang = (T3_t*v_tMax)/2;
    |     Dx = A_rect + A_triang;
    | else
    |     Dx = Ttot*Ttot*a_tMax/2;
    | end
    | 
    | if(x_fin>x_ini)
    |     X = x_fin - Dx;
    | else
    |     X = x_fin + Dx;
    | end
    | 
    | end
  function traslacion_calc(x_ini,x_fin):
    | function traslacion_calc(x_ini,x_fin)
    | 
    | dx = abs(x_fin - x_ini);    
    | 
    | t1x = (v_tMax - d_x_t)/a_tMax;    
    | t3x = abs(v_tMax/a_tMax);      
    | 
    | Dx1 = d_x_t * t1x + 0.5 * a_tMax * t1x*t1x;   
    | Dx3 = v_tMax * t3x - 0.5 * a_tMax * t3x*t3x;   
    | 
    | if ((Dx1 + Dx3) <= dx)
    |     xrest = dx - (Dx1 + Dx3);
    |     t2x = t1x + xrest / v_tMax;   
    |     vx = v_tMax;              
    |     tx_tot = t2x + t3x;       
    | else
    |     vx = sqrt(a_tMax * dx);   
    |     t3x = vx / a_tMax;       
    |     t2x = t3x - abs(d_x_t/a_tMax);
    |     tx_tot = t2x + t3x;       
    | end
    | 
    | end
  function trasladar(x_ini,x_fin,delta_t):
    | function trasladar(x_ini,x_fin,delta_t)
    | 
    | if(x_fin-x_ini>0)
    |     if (tx <= t2x)
    |         if (vel_t < vx)
    |             vel_t = vel_t + a_tMax * delta_t;
    |         else
    |             vel_t = vx;
    |         end
    |     else
    |         if (vel_t < 0)
    |             vel_t = 0;
    |         else
    |             vel_t = vel_t - a_tMax * delta_t;
    |         end
    |     end
    |     tx=tx+delta_t;
    |     
    | elseif(x_fin-x_ini<0)
    |     if (tx <= t2x)
    |         if (vel_t > -vx)
    |             vel_t = vel_t - a_tMax * delta_t;
    |         else
    |             vel_t = -vx;
    |         end
    |     else
    |         if (vel_t > 0)
    |             vel_t = 0;
    |         else
    |             vel_t = vel_t + a_tMax * delta_t;
    |         end
    |     end
    |     tx=tx+delta_t;
    |     
    | else
    |     vel_t = 0;
    | end
    | 
    | end
  function izaje_calc(y_ini,y_fin):
    | function izaje_calc(y_ini,y_fin)
    | 
    | dy = abs(y_fin - y_ini);    
    | 
    | t1y = (vel_hMax - d_x_h)/a_hMax;    
    | t3y = abs(vel_hMax/a_hMax);      
    | 
    | Dy1 = d_x_h * t1y + 0.5 * a_hMax * t1y*t1y;   
    | Dy3 =   vel_hMax * t3y - 0.5 * a_hMax * t3y*t3y;  
    | 
    | if ((Dy1 + Dy3) <= dy)
    |     yrest = dy - (Dy1 + Dy3); 
    |     t2y = t1y + yrest / vel_hMax;   
    |     vy = vel_hMax;                  
    |     ty_tot = t2y + t3y;       
    | else
    |     vy = sqrt(a_hMax * dy);   
    |     t3y = vy / a_hMax;        
    |     t2y = t3y - abs(d_x_h/a_hMax);
    |     ty_tot = t2y + t3y;       
    | end
    | 
    | end
  function izar(y_ini,y_fin,delta_t):
    | function izar(y_ini,y_fin,delta_t)
    | 
    | if(y_fin-y_ini>0)
    |     if (ty <= t2y)
    |         if (vel_h < vy)
    |             vel_h = vel_h + a_hMax * delta_t;
    |         else
    |             vel_h = vy;
    |         end
    |     else
    |         if (vel_h < 0)
    |             vel_h = 0;
    |         else
    |             vel_h = vel_h - a_hMax * delta_t;
    |         end
    |     end
    |     ty=ty+delta_t;
    |     
    | elseif(y_fin-y_ini<0)
    |     if (ty <= t2y)
    |         if (vel_h > -vy)
    |             vel_h = vel_h - a_hMax * delta_t;
    |         else
    |             vel_h = -vy;
    |         end
    |     else
    |         if (vel_h > 0)
    |             vel_h = 0;
    |         else
    |             vel_h = vel_h + a_hMax * delta_t;
    |         end
    |     end
    |     ty=ty+delta_t;
    |     
    | else
    |     vel_h = 0;
    | end
    | 
    | end
  function YmaxBarco = Ymax_b(Ycarga, carrilFin):
    | function YmaxBarco = Ymax_b(Ycarga, carrilFin)
    | 
    | offsetCarrilesBarco = 13; % Total carriles:32 - carriles en barco:18 - carril final:1 = 13
    | 
    | h_max = Y_sb;
    | for i=offsetCarrilesBarco+1:(carrilFin+offsetCarrilesBarco)
    |     if Ycarga(i)>=h_max
    |         h_max = Ycarga(i);
    |     end
    | end
    | YmaxBarco = h_max;
    | end

== matlab function ProyectoGlobal_AyCD_Cantu_LagoTejo/Nivel 2/MATLAB Function ==
  data: m_l input; l_h input; Kp output; Kd output; kd_bal input; kp_bal input
function [Kp,Kd] = fcn(m_l,l_h,kd_bal,kp_bal)
index_ml = ceil(m_l/100);
index_h = ceil(l_h/0.1);
if(index_ml <= 1)
   index_ml = 1; 
end

if(index_h <= 1)
   index_h = 1; 
end

if(index_ml >= 51)
   index_ml = 51; 
end

if(index_h >= 60)
   index_h = 60; 
end
Kd = kd_bal(index_ml,index_h);
Kp = kp_bal(index_ml,index_h);

end

== stateflow chart ProyectoGlobal_AyCD_Cantu_LagoTejo/Modelo Fisico Carro-Izaje-Carga/Chart ==
  settings: sampleTime=1e-3
  state CONTENEDOR_REAL [parallel]
    settings: executionOrder=1
    state CARGADO
      entry:
      h_c=H_c;
      M_cX = randi(M_cMax - M_cMin)+M_cMin;
      m_l_real=M_s+M_cX;
      %m_l_real=65000;
      %sobrePeso = 15000;
      %m_l_real=M_s+M_cX+sobrePeso;
    state DESCARGADO
      entry:
      m_l_real=M_s;
      h_c=0;
    CARGADO -> DESCARGADO : [cargado == 0]
    (default) -> DESCARGADO
    DESCARGADO -> CARGADO : [cargado == 1]
  state GRAFICA_PERFIL [parallel]
    entry:
    x_trm_plot=0;
    graficar=1;
    x_c=xc;
    y_c=yc;
    during:
    x_trm_plot=x_trm_plot+1e-3;
    if(change==1)
    y_c=yc_act;
    end
    if((x_trm_plot>0.998)&&(x_trm_plot<1.002))
    graficar=1;
    x_trm_plot=0;
    else
    graficar=0;
    end
    settings: executionOrder=2
  data: cargado input; M_s parameter; Mc_max local double size=1; sobrePeso local double size=1; Mc_min local double size=1; mRand local double size=1; h_c output double size=1; H_c parameter; x_aux local double size=[1 40]; y_c output size=[1 32]; change input; yc_act input size=[1 32]; graficar output size=1; x_trm_plot local; i local; yc2 local double; x_c output; xc parameter; yc parameter; M_cMin parameter; M_cMax parameter; M_cX local double size=1; m_l_real output

== stateflow chart ProyectoGlobal_AyCD_Cantu_LagoTejo/Nivel 0 ==
  settings: updateMethod=DISCRETE  sampleTime=1e-3
  state WATCHDOG3 [parallel]
    entry:
    cont_wd_0 = 0;
    cont_wd_1 = 0;
    during:
    if(ON_OFF==1)
    if (WD==0)
    cont_wd_1 = 0;
    cont_wd_0=cont_wd_0+1;
    if (cont_wd_0 > 51)
    EMER_WD=1;
    else
    EMER_WD=0;
    end
    elseif (WD==1)
    cont_wd_0 = 0;
    cont_wd_1=cont_wd_1+1;
    if (cont_wd_1 > 51)
    EMER_WD=1;
    else
    EMER_WD =0;
    end
    end
    end
    settings: executionOrder=2
  state CONTROL_DE_SEGURIDAD_NIVEL_0 [parallel]
    settings: executionOrder=1
    state NORMAL
      entry:
      EMER_WD=0;
      sistOK=1;
      BRK_hE=1;
      BRK_h = 1;
      BRK_t = 1;
      EMER_TOT=0;
      EMER_H=0;
      EMER_T=0;
    state EMERGENCIA_TOTAL
      during:
      sistOK = 0;
      manual_auto = 0;
      EMER_T = 1;
      EMER_H = 1;
      EMER_TOT=1;
      BRK_hE = 0;
      BRK_h = 0;
      BRK_t = 0;
    state EMERGENCIA_CARRO
      during:
      sistOK = 0;
      manual_auto = 0;
      EMER_T=1;
      BRK_t = 0;
    state EMERGENCIA_IZAJE
      during:
      sistOK = 0;
      manual_auto = 0;
      EMER_H=1;
      BRK_h = 0;
      BRK_hE = 0;
    state RESET
      entry:
      RESET_OK = 1;
    (default) -> NORMAL
    (junction 146) -> NORMAL
    NORMAL -> EMERGENCIA_CARRO [order 3] : [(fc_izq_ult)||(fc_der_ult)]
    NORMAL -> EMERGENCIA_IZAJE [order 1] : [(lim_v_h)||(fc_inf_ult)||(fc_sup_ult)]
    NORMAL -> EMERGENCIA_TOTAL [order 2] : [BTN_EMERGENCIA||EMER_WD]
    EMERGENCIA_CARRO -> RESET [order 1] : [fc_izq_ult == 0 && fc_der_ult == 0]
    EMERGENCIA_CARRO -> EMERGENCIA_TOTAL [order 3] : [EMER_WD || BTN_EMERGENCIA]
    EMERGENCIA_CARRO -> EMERGENCIA_TOTAL [order 2] : [fc_sup_ult  || fc_inf_ult || lim_v_h]
    EMERGENCIA_IZAJE -> EMERGENCIA_TOTAL [order 3] : [EMER_WD || BTN_EMERGENCIA]
    EMERGENCIA_IZAJE -> EMERGENCIA_TOTAL [order 2] : [[fc_izq_ult || fc_der_ult ]]
    EMERGENCIA_IZAJE -> RESET [order 1] : [lim_v_h == 0 && fc_sup_ult == 0 && fc_inf_ult == 0]
    EMERGENCIA_TOTAL -> RESET : [fc_izq_ult == 0 && fc_der_ult == 0 && fc_sup_ult == 0 && fc_inf_ult == 0 && lim_v_h==0 && BTN_EMERGENCIA==0 && EMER_WD==0]
    RESET -> (junction 146) : [(BTN_RESET)]
  (default) -> ?
  data: vel_t_on input; vel_h_on input; BTN_EMERGENCIA input; sistOK output; BRK_hE output; manual_auto output; BRK_h output; lim_v_h input; BRK_t output; F_hw input; ON_OFF input; MANUAL input; fc_izq_ult input; fc_der_ult input; fc_inf_ult input; fc_sup_ult input; WD input; cont_wd_1 local; cont_wd_0 local; EMER_WD output; EMER_T output; EMER_TOT output; EMER_H output; RESET_OK output; BTN_RESET input
